simulink model "MavicProComplete_oct22"  (R2019b)
settings: Solver=VariableStepAuto  StartTime=0  StopTime=1500  FixedStep=.01  MaxStep=10  MinStep=.01  RelTol=1e-4  EnableMultiTasking=on
InitFcn:
  | addpath params;
  | addpath fcns;
  | load batteryParams;
  | load motorParams;
  | load ukfBatteryParams;
  | load DJI.mat;
  | load DJIquadModel_X.mat;
model workspace (MAT data in the model file):
  Sig : Simulink.Signal (value not decoded)
values from neighbouring files (symbols this model uses):
  P = block.ContStates.Data(1)    [quadcopterDynamicsSFunctionMod.m]
  Phi = block.ContStates.Data(4)    [quadcopterDynamicsSFunctionMod.m]
  Psi = block.ContStates.Data(6)    [quadcopterDynamicsSFunctionMod.m]
  Q = block.ContStates.Data(2)    [quadcopterDynamicsSFunctionMod.m]
  R = block.ContStates.Data(3)    [quadcopterDynamicsSFunctionMod.m]
  The = block.ContStates.Data(5)    [quadcopterDynamicsSFunctionMod.m]
  Z = block.ContStates.Data(12)    [quadcopterDynamicsSFunctionMod.m]
undefined symbols (not defined in the file or in its folder): motorRes, quadModel
libraries: simulink x7, dspstat3 x5
(part 2 of 2)

== system MavicProComplete_oct22/Quadcopter/Powertrain/motorGroup/BLDC Motor1/throttle_fcn ==
  note: Output equals linearly scaled RPM
      | for given throttle input if throttle input >=Throttle Cuttoff (minThr)
      | else output is zero.
  In5 : Inport
  Vs : Inport  Port=2
  Gain : Gain  Gain=.01
  Minimum Throttle Cutoff : simulink/Logic and Bit Operations/Compare To Constant  relop=>=  const=5  OutDataTypeStr=uint8
  Product : Product
  Product2 : Product  OutDataTypeStr=double
  Out5 : Outport  VectorParamsAs1DForOutWhenUnconnected=off
  wires:
  Minimum Throttle Cutoff/1 -> Product/2
  Product/1 -> Out5/1
  In5/1 -> Gain/1, Minimum Throttle Cutoff/1
  Gain/1 -> Product2/2
  Product2/1 -> Product/1
  Vs/1 -> Product2/1

== system MavicProComplete_oct22/Quadcopter/Powertrain/motorGroup/BLDC Motor2/throttle_fcn ==
  note: Output equals linearly scaled RPM
      | for given throttle input if throttle input >=Throttle Cuttoff (minThr)
      | else output is zero.
  In5 : Inport
  Vs : Inport  Port=2
  Gain : Gain  Gain=.01
  Minimum Throttle Cutoff : simulink/Logic and Bit Operations/Compare To Constant  relop=>=  const=5  OutDataTypeStr=uint8
  Product : Product
  Product2 : Product  OutDataTypeStr=double
  Out5 : Outport  VectorParamsAs1DForOutWhenUnconnected=off
  wires:
  Minimum Throttle Cutoff/1 -> Product/2
  Product/1 -> Out5/1
  In5/1 -> Gain/1, Minimum Throttle Cutoff/1
  Gain/1 -> Product2/2
  Product2/1 -> Product/1
  Vs/1 -> Product2/1

== system MavicProComplete_oct22/Quadcopter/Powertrain/motorGroup/BLDC Motor3/throttle_fcn ==
  note: Output equals linearly scaled RPM
      | for given throttle input if throttle input >=Throttle Cuttoff (minThr)
      | else output is zero.
  In5 : Inport
  Vs : Inport  Port=2
  Gain : Gain  Gain=.01
  Minimum Throttle Cutoff : simulink/Logic and Bit Operations/Compare To Constant  relop=>=  const=5  OutDataTypeStr=uint8
  Product : Product
  Product2 : Product  OutDataTypeStr=double
  Out5 : Outport  VectorParamsAs1DForOutWhenUnconnected=off
  wires:
  Minimum Throttle Cutoff/1 -> Product/2
  Product/1 -> Out5/1
  In5/1 -> Gain/1, Minimum Throttle Cutoff/1
  Gain/1 -> Product2/2
  Product2/1 -> Product/1
  Vs/1 -> Product2/1

== system MavicProComplete_oct22/Quadcopter/Powertrain/motorGroup/BLDC Motor4/throttle_fcn ==
  note: Output equals linearly scaled RPM
      | for given throttle input if throttle input >=Throttle Cuttoff (minThr)
      | else output is zero.
  In5 : Inport
  Vs : Inport  Port=2
  Gain : Gain  Gain=.01
  Minimum Throttle Cutoff : simulink/Logic and Bit Operations/Compare To Constant  relop=>=  const=5  OutDataTypeStr=uint8
  Product : Product
  Product2 : Product  OutDataTypeStr=double
  Out5 : Outport  VectorParamsAs1DForOutWhenUnconnected=off
  wires:
  Minimum Throttle Cutoff/1 -> Product/2
  Product/1 -> Out5/1
  In5/1 -> Gain/1, Minimum Throttle Cutoff/1
  Gain/1 -> Product2/2
  Product2/1 -> Product/1
  Vs/1 -> Product2/1

== system MavicProComplete_oct22/Quadcopter/Powertrain/motorGroup/Subsystem/throttle_fcn ==
  note: Output equals linearly scaled RPM
      | for given throttle input if throttle input >=Throttle Cuttoff (minThr)
      | else output is zero.
  In5 : Inport
  Vs : Inport  Port=2
  Gain : Gain  Gain=.01
  Minimum Throttle Cutoff : simulink/Logic and Bit Operations/Compare To Constant  relop=>=  const=5  OutDataTypeStr=uint8
  Product : Product
  Product2 : Product  OutDataTypeStr=double
  Out5 : Outport  VectorParamsAs1DForOutWhenUnconnected=off
  wires:
  Minimum Throttle Cutoff/1 -> Product/2
  Product/1 -> Out5/1
  In5/1 -> Gain/1, Minimum Throttle Cutoff/1
  Gain/1 -> Product2/2
  Product2/1 -> Product/1
  Vs/1 -> Product2/1

== matlab function MavicProComplete_oct22/Quadcopter/Powertrain/3CellBattery/MATLAB Function1 ==
  settings: updateMethod=DISCRETE  sampleTime=.2
  data: mu input; y output; sigma input
function y = addNoise(mu, sigma)

y = normrnd(mu, sigma);

== matlab function MavicProComplete_oct22/Quadcopter/Powertrain/3CellBattery/MATLAB Function ==
  settings: updateMethod=DISCRETE  sampleTime=.2
  data: mu input; y output; sigma input
function y = addNoise(mu, sigma)

y = normrnd(mu, sigma);

== matlab function MavicProComplete_oct22/Quadcopter/Powertrain/motorGroup/Subsystem/MATLAB Function ==
  settings: updateMethod=DISCRETE  sampleTime=.2
  data: mu input; y output; sigma input
function y = addNoise(mu, sigma)

y = normrnd(mu, sigma);

== matlab function MavicProComplete_oct22/Quadcopter/wind_simulator/wind_and_gust/gust_to_drag ==
  data: gusts input; drag output
function drag = gust_to_drag(gusts)
%
% creates drag from wind gusts
%
% input: gusts (x,y,z)
%
% output: drag (x,y,z)
%

areas = [.0197 .0197 .0197*2*1.3];
drag = [0 0 0];
rho = 1.225;
coef_d = 1.0;

for i=1:3
    drag(i) = .5*rho*gusts(i)*areas(i)*coef_d;
    %if(gusts(i)>0)
    %    drag(i) = drag(i) * -1;
    %end   
end

== matlab function MavicProComplete_oct22/Quadcopter/Powertrain/motorGroup/Subsystem/MATLAB Function2 ==
  data: mu input; y output; sigma input
function y = addNoise(mu, sigma)

y = normrnd(mu, sigma);

== matlab function MavicProComplete_oct22/Quadcopter/Powertrain/motorGroup/BLDC Motor2/Propeller model  ==
  data: thrust output; torque output; rpm input
function [thrust,torque] = fcn(rpm)
% angular_velocity in rpm

%coefficient of thrust, empirically derived
coef_t = 2*(10^-15)*rpm^3 - 4*(10^-11)*rpm^2 + 3*(10^-7)*rpm + .1013;
%thrust = coef_t * density of air * velocity^2 * propeller diameter (m) ^4
thrust = coef_t*1.225*(rpm/60)^2*.2^4;
% empirically derived
torque = 4*(10^-14)*rpm^3 +  8*(10^-12)*rpm^2 + 3*(10^-6)*rpm;
end

== matlab function MavicProComplete_oct22/Quadcopter/Powertrain/motorGroup/BLDC Motor3/Propeller model  ==
  data: thrust output; torque output; rpm input
function [thrust,torque] = fcn(rpm)
% angular_velocity in rpm

%coefficient of thrust, empirically derived
coef_t = 2*(10^-15)*rpm^3 - 4*(10^-11)*rpm^2 + 3*(10^-7)*rpm + .1013;
%thrust = coef_t * density of air * velocity^2 * propeller diameter (m) ^4
thrust = coef_t*1.225*(rpm/60)^2*.2^4;
% empirically derived
torque = 4*(10^-14)*rpm^3 +  8*(10^-12)*rpm^2 + 3*(10^-6)*rpm;
end

== matlab function MavicProComplete_oct22/Quadcopter/Powertrain/motorGroup/BLDC Motor4/Propeller model  ==
  data: thrust output; torque output; rpm input
function [thrust,torque] = fcn(rpm)
% angular_velocity in rpm

%coefficient of thrust, empirically derived
coef_t = 2*(10^-15)*rpm^3 - 4*(10^-11)*rpm^2 + 3*(10^-7)*rpm + .1013;
%thrust = coef_t * density of air * velocity^2 * propeller diameter (m) ^4
thrust = coef_t*1.225*(rpm/60)^2*.2^4;
% empirically derived
torque = 4*(10^-14)*rpm^3 +  8*(10^-12)*rpm^2 + 3*(10^-6)*rpm;
end

== matlab function MavicProComplete_oct22/MATLAB Function ==
  data: pos input; y output; y input
function y = fcn(pos, y)

    if(pos >= 2000)
        y = y-.025;
    end

== matlab function MavicProComplete_oct22/Quadcopter/wind_simulator/wind_and_gust/gust_generator ==
  settings: updateMethod=DISCRETE
  data: period input; amplitude input; enabled input; gusts output; t input
function gusts = gust_generator(period, amplitude, enabled, t)

gusts = [0,0,0];
idx = 0;

if enabled == 1
    if mod(t,period) >= 1
        if rand > .8
            select = rand;
            if select < .3333
                idx = 1;
            elseif select > .6666
                idx = 3;
            else
                idx = 2;
            end % create a gust
            gusts(idx) = normrnd(0, amplitude);
        end
    end
end

== matlab function MavicProComplete_oct22/Quadcopter/Powertrain/motorGroup/BLDC Motor1/Propeller model  ==
  data: thrust output; torque output; rpm input
function [thrust,torque] = fcn(rpm)
% angular_velocity in rpm

%coefficient of thrust, empirically derived
coef_t = 2*(10^-15)*rpm^3 - 4*(10^-11)*rpm^2 + 3*(10^-7)*rpm + .1013;
%thrust = coef_t * density of air * velocity^2 * propeller diameter (m) ^4
thrust = coef_t*1.225*(rpm/60)^2*.2^4;
% empirically derived
torque = 4*(10^-14)*rpm^3 +  8*(10^-12)*rpm^2 + 3*(10^-6)*rpm;
end

== matlab function MavicProComplete_oct22/Quadcopter/wind_simulator/wind_and_gust/wind_generator  ==
  data: direction input; wind output; speed input; enabled input; t input
function wind = wind_generator(direction, speed, enabled, t)
%
% direction: 1 for tail wind, -1 for headwind
% speed: in m/s
%
wind = [0,0,0];

if enabled
    if direction ~= 1 && direction ~= -1
        error("direction should be 1 for tail wind or -1 for headwind");
    end
    if speed < 0 && speed > 5
        error("speed should be between 0 and 5");
    end
    wind(1) = 0;
    wind(2) = direction * speed;
    wind(3) = 0;
end
